simulink model "pilidar_main"  (R2017a)
settings: Solver=FixedStepAuto  StartTime=0.0  StopTime=inf  FixedStep=1/40  RelTol=1e-3
libraries: raspberrypilib x3, hdlsllib x1
settings Model: SimulationMode=external  Creator=WARA  LastModifiedBy=Vincent

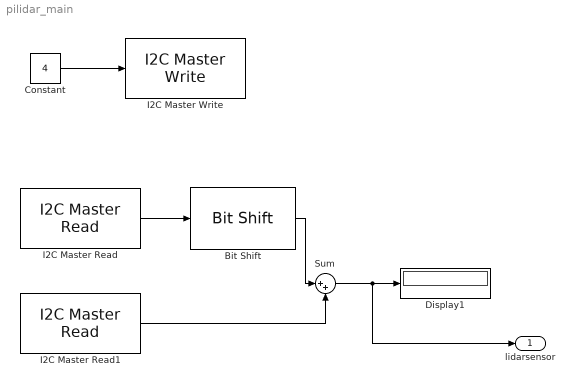
== system pilidar_main ==
  Bit Shift : hdlsllib/HDL Operations/Bit Shift  mode=Shift Left Logical  N=8
      settings: SourceProductName=HDL Coder  SourceProductBaseCode=HD
  Constant : Constant  Value=4
  Display1 : Display
  I2C Master Read : raspberrypilib/I2C Master Read  BoardProperty=Pi 3 Model B  Mode=Master  SlaveAddress=98  SlaveByteOrder=BigEndian  Direction=Receiver  RegisterAddressMode=on  RegisterAddress=143  SlaveDataType=uint8  DataLength=1  NoAck=off  RepeatedStart=off  OutputStatus=off  SampleTime=1/40
      settings: SourceProductName=Simulink Support Package for Raspberry Pi Hardware  SourceProductBaseCode=RASPPI
  I2C Master Read1 : raspberrypilib/I2C Master Read  BoardProperty=Pi 3 Model B  Mode=Master  SlaveAddress=98  SlaveByteOrder=BigEndian  Direction=Receiver  RegisterAddressMode=on  RegisterAddress=16  SlaveDataType=uint8  DataLength=1  NoAck=off  RepeatedStart=off  OutputStatus=off  SampleTime=1/40
      settings: SourceProductName=Simulink Support Package for Raspberry Pi Hardware  SourceProductBaseCode=RASPPI
  I2C Master Write : raspberrypilib/I2C Master Write  BoardProperty=Pi 3 Model B  Mode=Master  SlaveAddress=98  SlaveByteOrder=BigEndian  Direction=Transmitter  RegisterAddressMode=on  RegisterAddress=0  SlaveDataType=uint8  DataLength=1  NoAck=off  RepeatedStart=off  OutputStatus=off
      settings: SourceProductName=Simulink Support Package for Raspberry Pi Hardware  SourceProductBaseCode=RASPPI
  Sum : Sum  Inputs=|++
  lidarsensor : Outport  SampleTime=1/40
  wires:
  Bit Shift/1 -> Sum/1
  I2C Master Read/1 -> Bit Shift/1
  Constant/1 -> I2C Master Write/1
  Sum/1 -> lidarsensor/1, Display1/1
  I2C Master Read1/1 -> Sum/2
